simulink subsystem "LRLM_ECU"  (R2021a)
settings: Solver=VariableStepAuto  StartTime=0.0  StopTime=10.0  RelTol=1e-3
libraries: LRLM x4, BCM x2
settings Model: Creator=Sai229  LastModifiedBy=Sai229

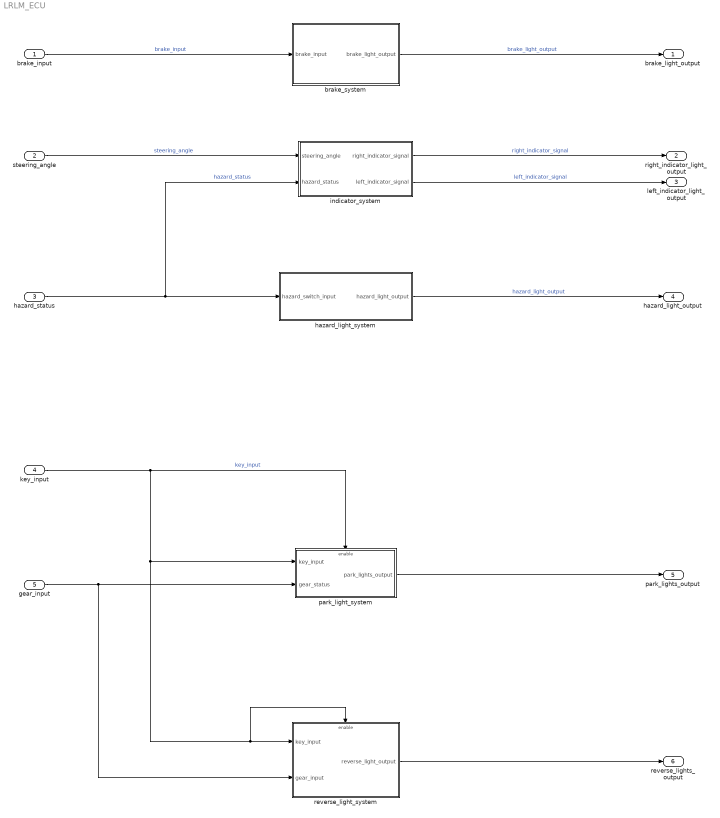
== system LRLM_ECU ==
  brake_input : Inport
  steering_angle : Inport  Port=2
  hazard_status : Inport  Port=3
  key_input : Inport  Port=4
  gear_input : Inport  Port=5
  brake_system : Subsystem
  hazard_light_system : Subsystem
  indicator_system : Subsystem
  park_light_system : Subsystem
  reverse_light_system : Subsystem
  brake_light_output : Outport
  right_indicator_light_output : Outport  Port=2
  left_indicator_light_output : Outport  Port=3
  hazard_light_output : Outport  Port=4
  park_lights_output : Outport  Port=5
  reverse_lights_output : Outport  Port=6
  wires:
  hazard_light_system/1(hazard_light_output) -> hazard_light_output/1  "hazard_light_output"
  gear_input/1 -> park_light_system/2(gear_status), reverse_light_system/2(gear_input)
  brake_input/1 -> brake_system/1(brake_input)  "brake_input"
  park_light_system/1(park_lights_output) -> park_lights_output/1
  key_input/1 -> park_light_system/Enable, park_light_system/1(key_input), reverse_light_system/1(key_input), reverse_light_system/Enable  "key_input"
  reverse_light_system/1(reverse_light_output) -> reverse_lights_output/1
  hazard_status/1 -> hazard_light_system/1(hazard_switch_input), indicator_system/2(hazard_status)  "hazard_status"
  indicator_system/2(left_indicator_signal) -> left_indicator_light_output/1  "left_indicator_signal"
  indicator_system/1(right_indicator_signal) -> right_indicator_light_output/1  "right_indicator_signal"
  steering_angle/1 -> indicator_system/1(steering_angle)  "steering_angle"
  brake_system/1(brake_light_output) -> brake_light_output/1  "brake_light_output"

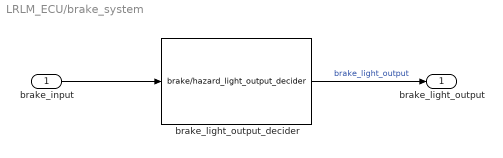
== system LRLM_ECU/brake_system ==
  brake_input : Inport
  brake_light_output_decider : LRLM/brake//hazard_light_output_decider
      settings: SourceProductName=LRLM Library
  brake_light_output : Outport
  wires:
  brake_light_output_decider/1 -> brake_light_output/1  "brake_light_output"
  brake_input/1 -> brake_light_output_decider/1

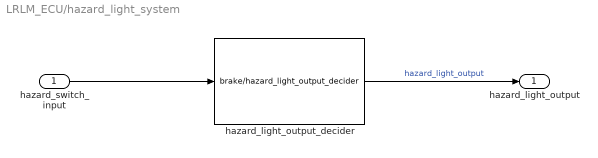
== system LRLM_ECU/hazard_light_system ==
  hazard_switch_input : Inport
  hazard_light_output_decider : LRLM/brake//hazard_light_output_decider
      settings: SourceProductName=LRLM Library
  hazard_light_output : Outport
  wires:
  hazard_light_output_decider/1 -> hazard_light_output/1  "hazard_light_output"
  hazard_switch_input/1 -> hazard_light_output_decider/1

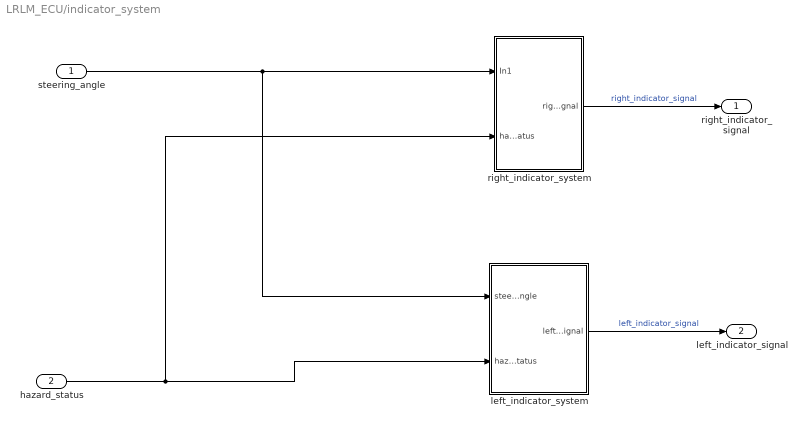
== system LRLM_ECU/indicator_system ==
  steering_angle : Inport
  hazard_status : Inport  Port=2
  left_indicator_system : Subsystem
  right_indicator_system : Subsystem
  right_indicator_signal : Outport
  left_indicator_signal : Outport  Port=2
  wires:
  steering_angle/1 -> right_indicator_system/1(In1), left_indicator_system/1(steering_angle)
  hazard_status/1 -> left_indicator_system/2(hazard_status), right_indicator_system/2(hazard_status)
  right_indicator_system/1(right_indicator_signal) -> right_indicator_signal/1  "right_indicator_signal"
  left_indicator_system/1(left_indicator_signal) -> left_indicator_signal/1  "left_indicator_signal"

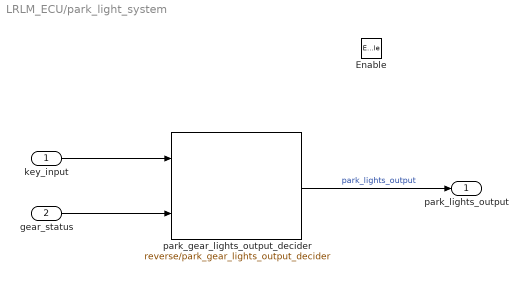
== system LRLM_ECU/park_light_system ==
  key_input : Inport
  gear_status : Inport  Port=2
  Enable : EnablePort  StatesWhenEnabling=reset
  park_gear_lights_output_decider : BCM/reverse//park_gear_lights_output_decider  gear_option=Neutral
      settings: SourceProductName=BCM Library
  park_lights_output : Outport
  wires:
  park_gear_lights_output_decider/1 -> park_lights_output/1  "park_lights_output"
  gear_status/1 -> park_gear_lights_output_decider/2
  key_input/1 -> park_gear_lights_output_decider/1

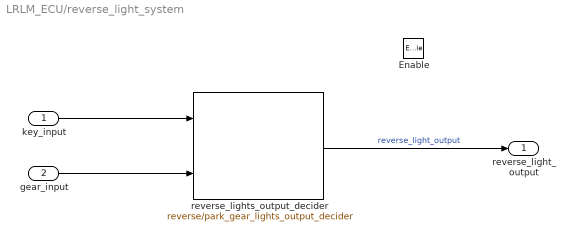
== system LRLM_ECU/reverse_light_system ==
  key_input : Inport
  gear_input : Inport  Port=2
  Enable : EnablePort  StatesWhenEnabling=reset
  reverse_lights_output_decider : BCM/reverse//park_gear_lights_output_decider  gear_option=Neutral
      settings: SourceProductName=BCM Library
  reverse_light_output : Outport
  wires:
  reverse_lights_output_decider/1 -> reverse_light_output/1  "reverse_light_output"
  gear_input/1 -> reverse_lights_output_decider/2
  key_input/1 -> reverse_lights_output_decider/1

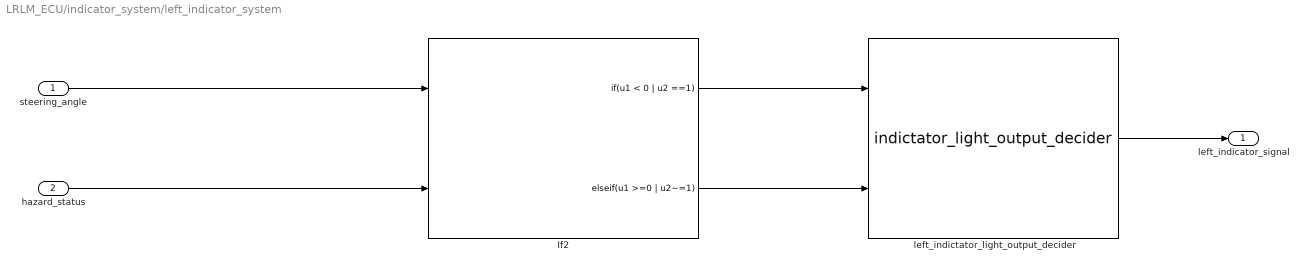
== system LRLM_ECU/indicator_system/left_indicator_system ==
  steering_angle : Inport
  hazard_status : Inport  Port=2
  If2 : If  NumInputs=2  IfExpression=u1 < 0 | u2 ==1  ElseIfExpressions=u1 >=0 | u2~=1  ShowElse=off
  left_indictator_light_output_decider : LRLM/indictator_light_output_decider
      settings: SourceProductName=LRLM Library
  left_indicator_signal : Outport
  wires:
  left_indictator_light_output_decider/1 -> left_indicator_signal/1
  If2/2 -> left_indictator_light_output_decider/2
  If2/1 -> left_indictator_light_output_decider/1
  steering_angle/1 -> If2/1
  hazard_status/1 -> If2/2

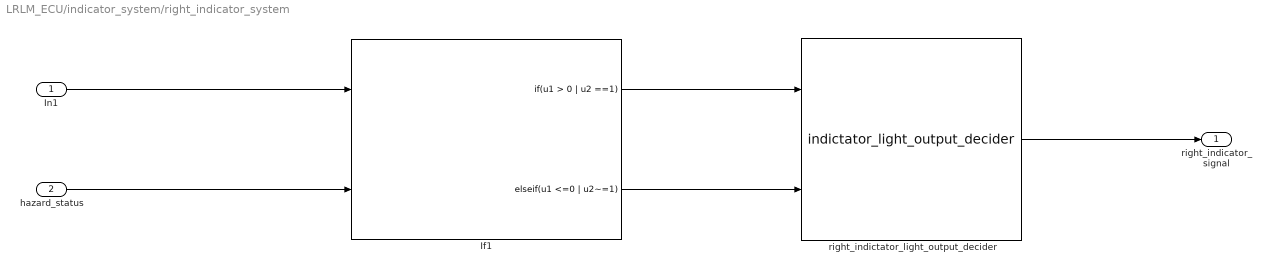
== system LRLM_ECU/indicator_system/right_indicator_system ==
  In1 : Inport
  hazard_status : Inport  Port=2
  If1 : If  NumInputs=2  IfExpression=u1 > 0 | u2 ==1  ElseIfExpressions=u1 <=0 | u2~=1  ShowElse=off
  right_indictator_light_output_decider : LRLM/indictator_light_output_decider
      settings: SourceProductName=LRLM Library
  right_indicator_signal : Outport
  wires:
  right_indictator_light_output_decider/1 -> right_indicator_signal/1
  If1/2 -> right_indictator_light_output_decider/2
  If1/1 -> right_indictator_light_output_decider/1
  In1/1 -> If1/1
  hazard_status/1 -> If1/2
